simulink model "MAT_SIM_SA"  (R2023b)
settings: Solver=ode45  StartTime=0.0  StopTime=10.0  RelTol=1e-3  EnableMultiTasking=on
values from neighbouring files (symbols this model uses):
  A = [       0,       1,         0,              -1 ... (first row only)    [MatLab_Simulink_Susp_ativa.m]
  B = [          0,      0 ... (first row only)    [MatLab_Simulink_Susp_ativa.m]
  C = [eye(4) ... (first row only)    [MatLab_Simulink_Susp_ativa.m]
  D = [zeros(4,2);0,0;0,1/M_s]    [MatLab_Simulink_Susp_ativa.m]
  K = [24.66 48.87 -0.47 3.68]    [MatLab_Simulink_Susp_ativa.m]
  Sel_Asfalto = 2    [MatLab_Simulink_Susp_ativa.m]
  Sel_Forca = 1    [MatLab_Simulink_Susp_ativa.m]
  Sel_Planta = 2    [MatLab_Simulink_Susp_ativa.m]
settings Model: Creator=Reginaldo Cardoso  LastModifiedBy=regin
settings SolverCC: AlgebraicLoopSolver=TrustRegion
settings DataIOCC: LimitDataPoints=on  SaveFormat=Array  ReturnWorkspaceOutputs=off
settings OptimizationCC: ExpressionDepthLimit=2147483647  LifeSpan=inf
settings DebuggingCC: AlgebraicLoopMsg=none  UnderspecifiedInitializationDetection=Classic  MergeDetectMultiDrivingBlocksExec=none  UnconnectedInputMsg=warning  UnconnectedOutputMsg=warning  UnconnectedLineMsg=warning  StateNameClashWarn=warning  SFUnexpectedBacktrackingDiag=warning  SFNoUnconditionalDefaultTransitionDiag=warning  SFExecutionAtInitializationDiag=none  ArithmeticOperatorsInVariantConditions=warning
settings HardwareCC: ProdBitPerPointer=32  ProdBitPerSizeT=32  ProdBitPerPtrDiffT=32  ProdLargestAtomicFloat=None  ProdIntDivRoundTo=Undefined  ProdEndianess=Unspecified  ProdWordSize=32  ProdHWDeviceType=32-bit Generic
settings ModelReferenceCC: PropagateSignalLabelsOutOfModel=off
settings SFSimCC: SimUseLocalCustomCode=off  CustomCodeUndefinedFunction=UseInterfaceOnly
settings RTWCC: RTWUseLocalCustomCode=off
settings CodeAppCC: StateflowObjectComments=on
settings GRTTargetCC: TargetLangStandard=C89/C90 (ANSI)
settings ConfigComp: CovMetricSettings=dw  CovSaveCumulativeToWorkspaceVar=on  CovSaveSingleToWorkspaceVar=on  CovExternalEMLEnable=off

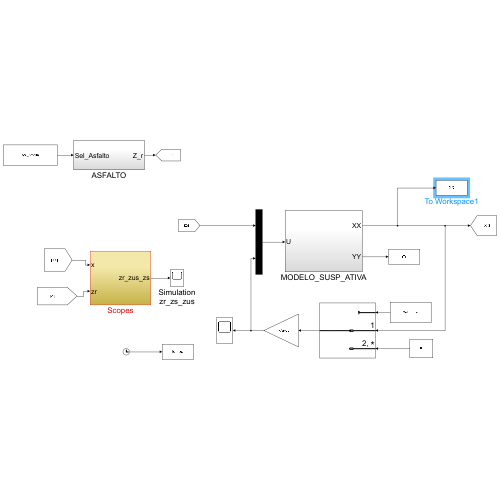
[thumbnail: Simulink's stored preview of the top-level diagram]
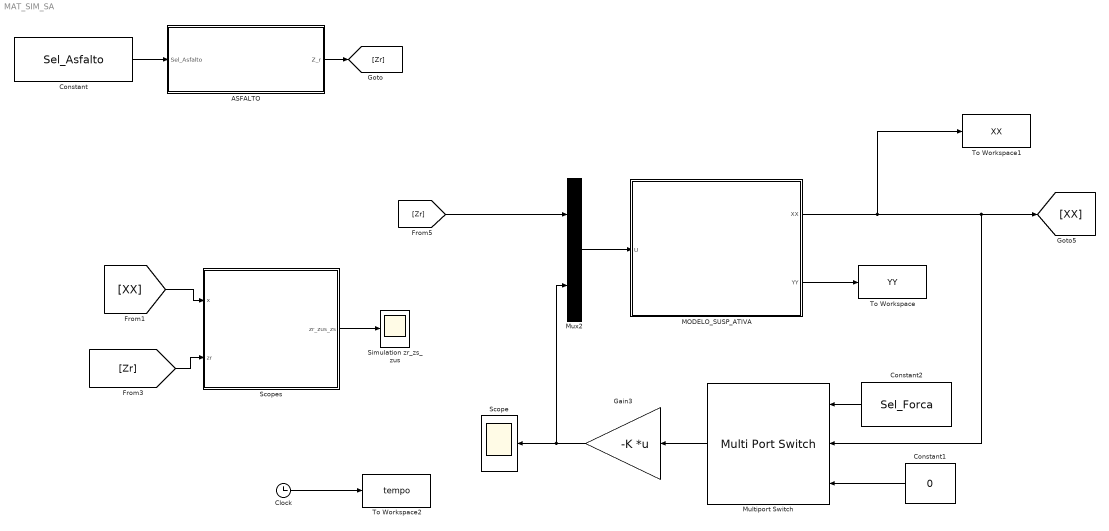
== system MAT_SIM_SA ==
  ASFALTO : Subsystem
  Clock : Clock
  Constant : Constant  Value=Sel_Asfalto
  Constant1 : Constant  Value=0
  Constant2 : Constant  Value=Sel_Forca
  Gain3 : Gain  Gain=-K  Multiplication=Matrix(K*u) (u vector)
  MODELO_SUSP_ATIVA : Subsystem
  Multiport Switch : MultiPortSwitch  Inputs=2  DiagnosticForDefault=None  SaturateOnIntegerOverflow=off  InputSameDT=off
  Mux2 : Mux  Inputs=2
  Scope : Scope
  Scopes : Subsystem
  Simulation zr_zs_zus : Scope
  To Workspace : ToWorkspace  VariableName=YY  SampleTime=-1
  To Workspace1 : ToWorkspace  VariableName=XX  SampleTime=-1
  To Workspace2 : ToWorkspace  VariableName=tempo  SampleTime=-1
  wires:
  [Zr] -> Mux2/1
  Gain3/1 -> Scope/1, Mux2/2
  ASFALTO/1(Z_r) -> [Zr]
  Constant/1 -> ASFALTO/1(Sel_Asfalto)
  [XX] -> Scopes/1(x)
  [Zr] -> Scopes/2(zr)
  Scopes/1(zr_zus_zs) -> Simulation zr_zs_zus/1
  Mux2/1 -> MODELO_SUSP_ATIVA/1(U)
  MODELO_SUSP_ATIVA/1(XX) -> To Workspace1/1, Multiport Switch/2, [XX]
  MODELO_SUSP_ATIVA/2(YY) -> To Workspace/1
  Multiport Switch/1 -> Gain3/1
  Constant1/1 -> Multiport Switch/3
  Constant2/1 -> Multiport Switch/1
  Clock/1 -> To Workspace2/1

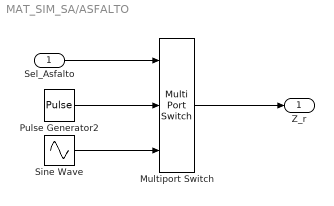
== system MAT_SIM_SA/ASFALTO ==
  Sel_Asfalto : Inport
  Multiport Switch : MultiPortSwitch  Inputs=2  DiagnosticForDefault=None  SaturateOnIntegerOverflow=off  InputSameDT=off
  Pulse Generator2 : DiscretePulseGenerator  PulseType=Time based  Amplitude=0.02  Period=3  PulseWidth=50  PhaseDelay=.1
  Sine Wave : Sin  Amplitude=0.02  Frequency=pi/0.3  SampleTime=0
  Z_r : Outport
  wires:
  Multiport Switch/1 -> Z_r/1
  Pulse Generator2/1 -> Multiport Switch/2
  Sine Wave/1 -> Multiport Switch/3
  Sel_Asfalto/1 -> Multiport Switch/1

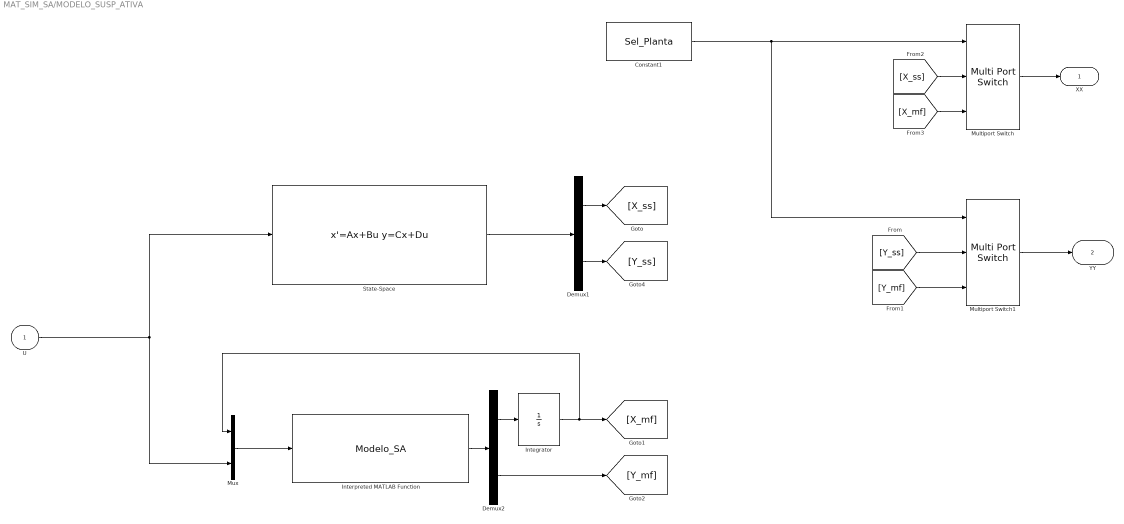
== system MAT_SIM_SA/MODELO_SUSP_ATIVA ==
  U : Inport
  Constant1 : Constant  Value=Sel_Planta
  Demux1 : Demux  Outputs=[4;2]
  Demux2 : Demux  Outputs=[4;2]
  Integrator : Integrator
  Interpreted MATLAB Function : MATLABFcn  MATLABFcn=Modelo_SA  OutputDimensions=6
  Multiport Switch : MultiPortSwitch  Inputs=2  DiagnosticForDefault=None  SaturateOnIntegerOverflow=off  InputSameDT=off
  Multiport Switch1 : MultiPortSwitch  Inputs=2  DiagnosticForDefault=None  SaturateOnIntegerOverflow=off  InputSameDT=off
  Mux : Mux  Inputs=[4;2]
  State-Space : StateSpace  A=A  B=B  C=C  D=D  InitialCondition=0
  XX : Outport
  YY : Outport  Port=2
  wires:
  U/1 -> State-Space/1, Mux/2
  Mux/1 -> Interpreted MATLAB Function/1
  Interpreted MATLAB Function/1 -> Demux2/1
  Demux2/1 -> Integrator/1
  Integrator/1 -> [X_mf], Mux/1
  State-Space/1 -> Demux1/1
  Constant1/1 -> Multiport Switch/1, Multiport Switch1/1
  Demux2/2 -> [Y_mf]
  Demux1/2 -> [Y_ss]
  Demux1/1 -> [X_ss]
  [X_ss] -> Multiport Switch/2
  [X_mf] -> Multiport Switch/3
  [Y_ss] -> Multiport Switch1/2
  [Y_mf] -> Multiport Switch1/3
  Multiport Switch1/1 -> YY/1
  Multiport Switch/1 -> XX/1

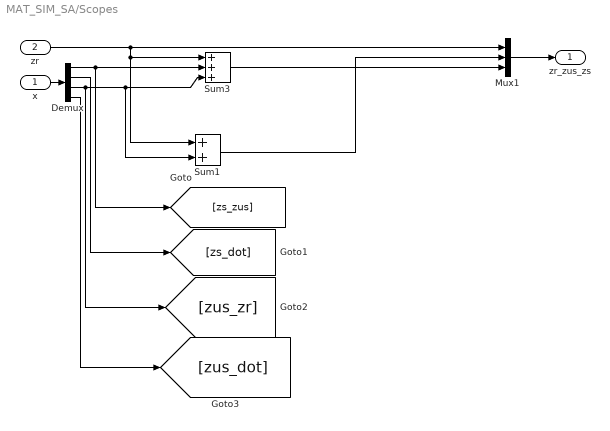
== system MAT_SIM_SA/Scopes ==
  x : Inport
  zr : Inport  Port=2
  Demux : Demux
  Mux1 : Mux  Inputs=3
  Sum1 : Sum  Inputs=2  InputSameDT=on  SaturateOnIntegerOverflow=on  OutDataTypeStr=Inherit: Same as first input
  Sum3 : Sum  Inputs=3  InputSameDT=on  SaturateOnIntegerOverflow=on  OutDataTypeStr=Inherit: Same as first input
  zr_zus_zs : Outport
  wires:
  Demux/1 -> Sum3/2, [zs_zus]
  Demux/3 -> Sum3/3, Sum1/2, [zus_zr]
  zr/1 -> Mux1/1, Sum3/1, Sum1/1
  x/1 -> Demux/1
  Demux/2 -> [zs_dot]
  Demux/4 -> [zus_dot]
  Sum1/1 -> Mux1/2
  Sum3/1 -> Mux1/3
  Mux1/1 -> zr_zus_zs/1
